simulink model "DDC_FIXED_POINT_2018a"  (R2018a)
settings: Solver=FixedStepDiscrete  StartTime=0.0  StopTime=2  FixedStep=1/69.333e3  RelTol=1e-3
PreLoadFcn:
  | gsmcoeffs
libraries: dspmlti4 x10, dspobslib x2, dspsrcs4 x1, dspmathops x1
settings Model: Creator=denis  LastModifiedBy=sda
settings DataIOCC: LimitDataPoints=on  SaveFormat=Array
settings OptimizationCC: LifeSpan=inf
settings DebuggingCC: SolverPrmCheckMsg=warning  SFUnexpectedBacktrackingDiag=warning  SFNoUnconditionalDefaultTransitionDiag=warning  SFExecutionAtInitializationDiag=none
settings HardwareCC: ProdBitPerPointer=32  ProdBitPerSizeT=32  ProdBitPerPtrDiffT=32  ProdLargestAtomicFloat=None  ProdIntDivRoundTo=Undefined  ProdEndianess=Unspecified  ProdWordSize=32  ProdHWDeviceType=ASIC/FPGA->ASIC/FPGA  TargetBitPerLong=64  TargetBitPerPointer=64  TargetBitPerSizeT=64  TargetBitPerPtrDiffT=64  TargetLongLongMode=on  TargetIntDivRoundTo=Zero  TargetEndianess=LittleEndian  TargetWordSize=64  TargetHWDeviceType=Custom Processor->MATLAB Host Computer  ProdEqTarget=off
settings ModelReferenceCC: PropagateSignalLabelsOutOfModel=off
settings CodeAppCC: StateflowObjectComments=on
settings GRTTargetCC: TargetLangStandard=C89/C90 (ANSI)
settings ConfigComp: CovMetricSettings=dw  CovHtmlReporting=on  CovSaveCumulativeToWorkspaceVar=on  CovSaveSingleToWorkspaceVar=on  CovExternalEMLEnable=off

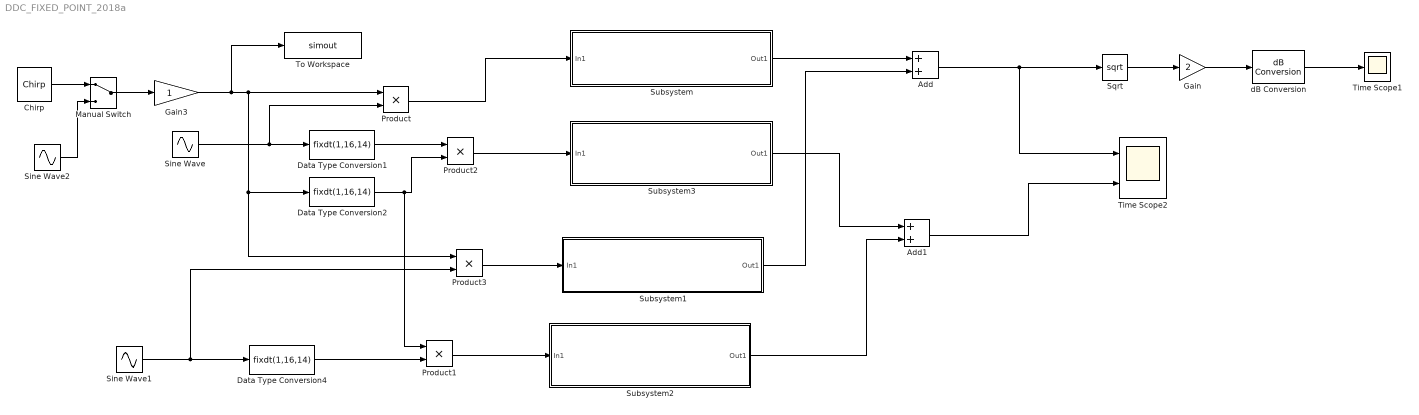
== system DDC_FIXED_POINT_2018a ==
  Add : Sum
  Add1 : Sum  OutDataTypeStr=fixdt(1,16,14)
  Chirp : dspsrcs4/Chirp  sweep=Linear  mode=Unidirectional  f0=13000  f1=16000  t1=2  Tsweep=4  phase=0  Ts=1/69.333e3  spf=1  datatype=Double  OutputFrames=on
  Data Type Conversion1 : DataTypeConversion  OutDataTypeStr=fixdt(1,16,14)
  Data Type Conversion2 : DataTypeConversion  OutDataTypeStr=fixdt(1,16,14)
  Data Type Conversion4 : DataTypeConversion  OutDataTypeStr=fixdt(1,16,14)
  Gain : Gain  Gain=2
  Gain3 : Gain
  Manual Switch : ManualSwitch
  Product : Product  OutMin=0  OutMax=1  OutDataTypeStr=double
  Product1 : Product  OutMin=0  OutMax=1  OutDataTypeStr=fixdt(1,16,14)
  Product2 : Product  OutMin=0  OutMax=1  OutDataTypeStr=fixdt(1,16,14)
  Product3 : Product  OutMin=0  OutMax=1  OutDataTypeStr=double
  Sine Wave : Sin  Frequency=14.44e3*2*pi  SampleTime=1/69.333e3
  Sine Wave1 : Sin  Frequency=14.44e3*2*pi  Phase=pi/2  SampleTime=1/69.333e3
  Sine Wave2 : Sin  Frequency=14.44e3*2*pi  Phase=pi/2  SampleTime=1/69.333e3
  Sqrt : Sqrt  SaturateOnIntegerOverflow=on
  Subsystem : Subsystem
  Subsystem1 : Subsystem
  Subsystem2 : Subsystem
  Subsystem3 : Subsystem
  Time Scope1 : Scope
  Time Scope2 : Scope  NumInputPorts=2
  To Workspace : ToWorkspace  VariableName=simout  SampleTime=-1
      settings: Save2DSignal=2-D array (concatenate along first dimension)
  dB Conversion : dspmathops/dB Conversion  dBtype=dB  intype=Amplitude  R=1  fuzz=on
  wires:
  Sine Wave/1 -> Data Type Conversion1/1, Product/2
  Sqrt/1 -> Gain/1
  Gain/1 -> dB Conversion/1
  dB Conversion/1 -> Time Scope1/1
  Chirp/1 -> Manual Switch/1
  Manual Switch/1 -> Gain3/1
  Sine Wave2/1 -> Manual Switch/2
  Product/1 -> Subsystem/1(In1)
  Subsystem/1(Out1) -> Add/1
  Sine Wave1/1 -> Product3/2, Data Type Conversion4/1
  Data Type Conversion4/1 -> Product1/2
  Subsystem2/1(Out1) -> Add1/2
  Subsystem3/1(Out1) -> Add1/1
  Subsystem1/1(Out1) -> Add/2
  Add1/1 -> Time Scope2/2
  Gain3/1 -> To Workspace/1, Product3/1, Data Type Conversion2/1, Product/1
  Product2/1 -> Subsystem3/1(In1)
  Data Type Conversion1/1 -> Product2/1
  Data Type Conversion2/1 -> Product1/1, Product2/2
  Product3/1 -> Subsystem1/1(In1)
  Product1/1 -> Subsystem2/1(In1)
  Add/1 -> Time Scope2/1, Sqrt/1

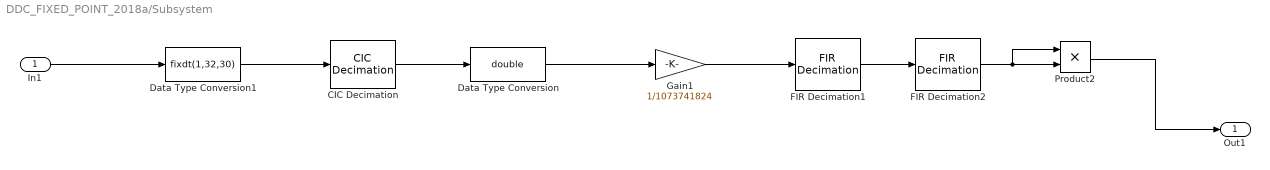
== system DDC_FIXED_POINT_2018a/Subsystem ==
  In1 : Inport
  CIC Decimation : dspobslib/CIC Decimation  filtFrom=Dialog  filtobj=Hm_decim  ftype=Decimator  R=64  M=1  N=5  filterInternals=Full precision  BPS=[16 16 16 16]  FLPS=0  outputWordLength=20  outputFracLength=0  launchFVT=off  framing=Maintain input frame rate  RateOptions=Allow multirate processing
      settings: SourceProductBaseCode=DS
  Data Type Conversion : DataTypeConversion  OutDataTypeStr=double
  Data Type Conversion1 : DataTypeConversion  OutDataTypeStr=fixdt(1,32,30)
  FIR Decimation1 : dspmlti4/FIR Decimation  FilterSource=Dialog parameters  h=cfir  D=2  filtStruct=Direct form  FilterObject=Hm_firdecim  InputProcessing=Columns as channels (frame based)  framing=Allow multirate processing  inputOffset=0  outputBufInitCond=0  roundingMode=Floor  overflowMode=off  firstCoeffDataTypeStr=Inherit: Same word length as input  firstCoeffMin=[]  firstCoeffMax=16  firstCoeffLastDataTypeStr=Inherit: Same word length as input  outputMode=Binary point scaling  outputWordLength=20  outputFracLength=12  outputDataTypeStr=fixdt(1,20,12)  outputMin=[]  outputMax=[]  outputLastDataTypeStr=fixdt(1,20,12)
  FIR Decimation2 : dspmlti4/FIR Decimation  FilterSource=Dialog parameters  h=pfir  D=2  filtStruct=Direct form  FilterObject=Hm_firdecim  InputProcessing=Columns as channels (frame based)  framing=Allow multirate processing  inputOffset=0  outputBufInitCond=0  roundingMode=Floor  overflowMode=off  firstCoeffDataTypeStr=Inherit: Same word length as input  firstCoeffMin=[]  firstCoeffMax=16  firstCoeffLastDataTypeStr=Inherit: Same word length as input  outputMode=Binary point scaling  outputWordLength=20  outputFracLength=12  outputDataTypeStr=fixdt(1,20,12)  outputMin=[]  outputMax=[]  outputLastDataTypeStr=fixdt(1,20,12)
  Gain1 : Gain  Gain=1/1073741824
  Product2 : Product  OutMin=0  OutMax=1  OutDataTypeStr=double
  Out1 : Outport
  wires:
  CIC Decimation/1 -> Data Type Conversion/1
  Product2/1 -> Out1/1
  Data Type Conversion/1 -> Gain1/1
  FIR Decimation1/1 -> FIR Decimation2/1
  Gain1/1 -> FIR Decimation1/1
  FIR Decimation2/1 -> Product2/1, Product2/2
  Data Type Conversion1/1 -> CIC Decimation/1
  In1/1 -> Data Type Conversion1/1

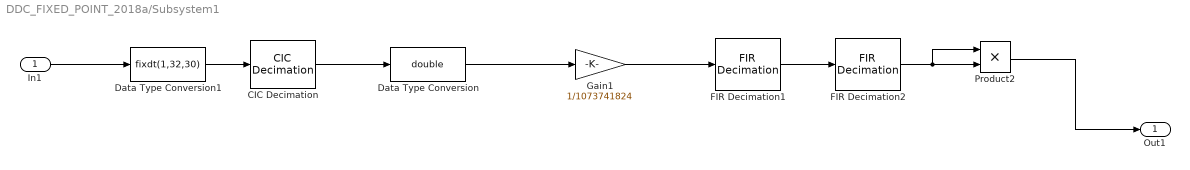
== system DDC_FIXED_POINT_2018a/Subsystem1 ==
  In1 : Inport
  CIC Decimation : dspobslib/CIC Decimation  filtFrom=Dialog  filtobj=Hm_decim  ftype=Decimator  R=64  M=1  N=5  filterInternals=Full precision  BPS=[16 16 16 16]  FLPS=0  outputWordLength=20  outputFracLength=0  launchFVT=off  framing=Maintain input frame rate  RateOptions=Allow multirate processing
      settings: SourceProductBaseCode=DS
  Data Type Conversion : DataTypeConversion  OutDataTypeStr=double
  Data Type Conversion1 : DataTypeConversion  OutDataTypeStr=fixdt(1,32,30)
  FIR Decimation1 : dspmlti4/FIR Decimation  FilterSource=Dialog parameters  h=cfir  D=2  filtStruct=Direct form  FilterObject=Hm_firdecim  InputProcessing=Columns as channels (frame based)  framing=Allow multirate processing  inputOffset=0  outputBufInitCond=0  roundingMode=Floor  overflowMode=off  firstCoeffDataTypeStr=Inherit: Same word length as input  firstCoeffMin=[]  firstCoeffMax=16  firstCoeffLastDataTypeStr=Inherit: Same word length as input  outputMode=Binary point scaling  outputWordLength=20  outputFracLength=12  outputDataTypeStr=fixdt(1,20,12)  outputMin=[]  outputMax=[]  outputLastDataTypeStr=fixdt(1,20,12)
  FIR Decimation2 : dspmlti4/FIR Decimation  FilterSource=Dialog parameters  h=pfir  D=2  filtStruct=Direct form  FilterObject=Hm_firdecim  InputProcessing=Columns as channels (frame based)  framing=Allow multirate processing  inputOffset=0  outputBufInitCond=0  roundingMode=Floor  overflowMode=off  firstCoeffDataTypeStr=Inherit: Same word length as input  firstCoeffMin=[]  firstCoeffMax=16  firstCoeffLastDataTypeStr=Inherit: Same word length as input  outputMode=Binary point scaling  outputWordLength=20  outputFracLength=12  outputDataTypeStr=fixdt(1,20,12)  outputMin=[]  outputMax=[]  outputLastDataTypeStr=fixdt(1,20,12)
  Gain1 : Gain  Gain=1/1073741824
  Product2 : Product  OutMin=0  OutMax=1  OutDataTypeStr=double
  Out1 : Outport
  wires:
  CIC Decimation/1 -> Data Type Conversion/1
  In1/1 -> Data Type Conversion1/1
  Product2/1 -> Out1/1
  Data Type Conversion/1 -> Gain1/1
  FIR Decimation1/1 -> FIR Decimation2/1
  Gain1/1 -> FIR Decimation1/1
  FIR Decimation2/1 -> Product2/1, Product2/2
  Data Type Conversion1/1 -> CIC Decimation/1

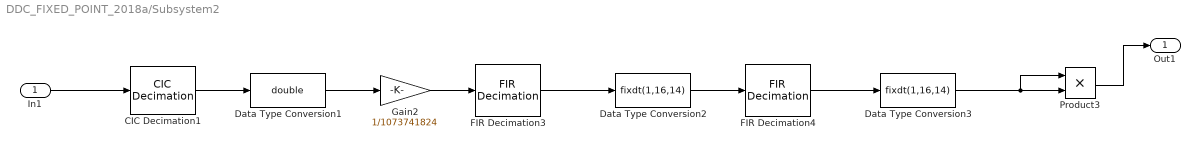
== system DDC_FIXED_POINT_2018a/Subsystem2 ==
  In1 : Inport
  CIC Decimation1 : dspmlti4/CIC Decimation  filtFrom=Dialog  filtobj=Hm_decim  ftype=Decimator  R=64  M=1  N=5  filterInternals=Full precision  BPS=[16 16 16 16]  FLPS=0  outputWordLength=20  outputFracLength=0  launchFVT=off  framing=Maintain input frame rate  RateOptions=Allow multirate processing
      settings: SourceProductBaseCode=DS
  Data Type Conversion1 : DataTypeConversion  OutDataTypeStr=double
  Data Type Conversion2 : DataTypeConversion  OutDataTypeStr=fixdt(1,16,14)
  Data Type Conversion3 : DataTypeConversion  OutDataTypeStr=fixdt(1,16,14)
  FIR Decimation3 : dspmlti4/FIR Decimation  FilterSource=Dialog parameters  h=cfir  D=2  filtStruct=Direct form  FilterObject=Hm_firdecim  InputProcessing=Columns as channels (frame based)  framing=Allow multirate processing  inputOffset=0  outputBufInitCond=0  roundingMode=Floor  overflowMode=off  firstCoeffMode=Binary point scaling  firstCoeffWordLength=16  firstCoeffFracLength=16  firstCoeffDataTypeStr=fixdt(1,16,16)  firstCoeffMin=[]  firstCoeffMax=0.49  firstCoeffLastDataTypeStr=fixdt(1,16,16)  outputDataTypeStr=Inherit: Same as accumulator  outputMin=[]  outputMax=[]  outputLastDataTypeStr=Inherit: Same as accumulator
  FIR Decimation4 : dspmlti4/FIR Decimation  FilterSource=Dialog parameters  h=pfir  D=2  filtStruct=Direct form  FilterObject=Hm_firdecim  InputProcessing=Columns as channels (frame based)  framing=Allow multirate processing  inputOffset=0  outputBufInitCond=0  roundingMode=Floor  overflowMode=off  firstCoeffMode=Binary point scaling  firstCoeffWordLength=16  firstCoeffFracLength=16  firstCoeffDataTypeStr=fixdt(1,16,16)  firstCoeffMin=[]  firstCoeffMax=0.49  firstCoeffLastDataTypeStr=fixdt(1,16,16)  outputDataTypeStr=Inherit: Same as accumulator  outputMin=[]  outputMax=[]  outputLastDataTypeStr=Inherit: Same as accumulator
  Gain2 : Gain  Gain=1/1073741824  OutDataTypeStr=fixdt(1,16,14)  RndMeth=Simplest
  Product3 : Product  OutMin=0  OutMax=1  OutDataTypeStr=fixdt(1,16,14)
  Out1 : Outport  VectorParamsAs1DForOutWhenUnconnected=on
  wires:
  Gain2/1 -> FIR Decimation3/1
  FIR Decimation4/1 -> Data Type Conversion3/1
  FIR Decimation3/1 -> Data Type Conversion2/1
  Data Type Conversion1/1 -> Gain2/1
  CIC Decimation1/1 -> Data Type Conversion1/1
  Data Type Conversion3/1 -> Product3/2, Product3/1
  Product3/1 -> Out1/1
  Data Type Conversion2/1 -> FIR Decimation4/1
  In1/1 -> CIC Decimation1/1

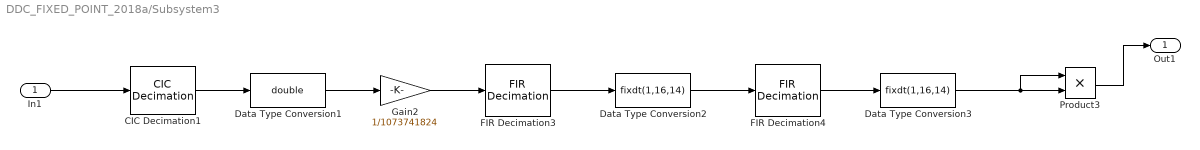
== system DDC_FIXED_POINT_2018a/Subsystem3 ==
  In1 : Inport
  CIC Decimation1 : dspmlti4/CIC Decimation  filtFrom=Dialog  filtobj=Hm_decim  ftype=Decimator  R=64  M=1  N=5  filterInternals=Full precision  BPS=[16 16 16 16]  FLPS=0  outputWordLength=20  outputFracLength=0  launchFVT=off  framing=Maintain input frame rate  RateOptions=Allow multirate processing
      settings: SourceProductBaseCode=DS
  Data Type Conversion1 : DataTypeConversion  OutDataTypeStr=double
  Data Type Conversion2 : DataTypeConversion  OutDataTypeStr=fixdt(1,16,14)
  Data Type Conversion3 : DataTypeConversion  OutDataTypeStr=fixdt(1,16,14)
  FIR Decimation3 : dspmlti4/FIR Decimation  FilterSource=Dialog parameters  h=cfir  D=2  filtStruct=Direct form  FilterObject=Hm_firdecim  InputProcessing=Columns as channels (frame based)  framing=Allow multirate processing  inputOffset=0  outputBufInitCond=0  roundingMode=Floor  overflowMode=off  firstCoeffMode=Binary point scaling  firstCoeffWordLength=16  firstCoeffFracLength=16  firstCoeffDataTypeStr=fixdt(1,16,16)  firstCoeffMin=[]  firstCoeffMax=0.49  firstCoeffLastDataTypeStr=fixdt(1,16,16)  outputDataTypeStr=Inherit: Same as accumulator  outputMin=[]  outputMax=[]  outputLastDataTypeStr=Inherit: Same as accumulator
  FIR Decimation4 : dspmlti4/FIR Decimation  FilterSource=Dialog parameters  h=pfir  D=2  filtStruct=Direct form  FilterObject=Hm_firdecim  InputProcessing=Columns as channels (frame based)  framing=Allow multirate processing  inputOffset=0  outputBufInitCond=0  roundingMode=Floor  overflowMode=off  firstCoeffMode=Binary point scaling  firstCoeffWordLength=16  firstCoeffFracLength=16  firstCoeffDataTypeStr=fixdt(1,16,16)  firstCoeffMin=[]  firstCoeffMax=0.49  firstCoeffLastDataTypeStr=fixdt(1,16,16)  outputDataTypeStr=Inherit: Same as accumulator  outputMin=[]  outputMax=[]  outputLastDataTypeStr=Inherit: Same as accumulator
  Gain2 : Gain  Gain=1/1073741824  OutDataTypeStr=fixdt(1,16,14)  RndMeth=Simplest
  Product3 : Product  OutMin=0  OutMax=1  OutDataTypeStr=fixdt(1,16,14)
  Out1 : Outport  VectorParamsAs1DForOutWhenUnconnected=on
  wires:
  Gain2/1 -> FIR Decimation3/1
  FIR Decimation4/1 -> Data Type Conversion3/1
  FIR Decimation3/1 -> Data Type Conversion2/1
  Data Type Conversion1/1 -> Gain2/1
  CIC Decimation1/1 -> Data Type Conversion1/1
  Data Type Conversion3/1 -> Product3/2, Product3/1
  Product3/1 -> Out1/1
  Data Type Conversion2/1 -> FIR Decimation4/1
  In1/1 -> CIC Decimation1/1
